simulink model "simulazione_006_s"  (R2016b)
settings: Solver=ode4  StartTime=0.0  StopTime=t_sim  FixedStep=step  RelTol=1e-3
values from neighbouring files (symbols this model uses):
  motion_time = 5    [simulazione_006_init.m]
  movement_lower_limit = -movement_upper_limit    [simulazione_006_init.m]
  movement_upper_limit = [2*pi; 2*pi; 2*pi; 2*pi; 2*pi; 2*pi]    [simulazione_006_init.m]
  p_init = direct_kinematic(q_init)    [simulazione_006_init.m]
  q_init = [pi/2; pi/3; -pi/9; pi/3; pi/5; pi/8]    [simulazione_006_init.m]
  radius = 0.1    [simulazione_006_init.m]
  ref_pulse = 2 * pi * frequency    (= 0.628318530718)    [simulazione_006_init.m]
  velocity_lower_limit = -velocity_upper_limit    [simulazione_006_init.m]
  velocity_upper_limit = [2*pi/3; 2*pi/3; pi; pi; pi; pi]    [simulazione_006_init.m]
settings Model: Creator=IBM  LastModifiedBy=IBM

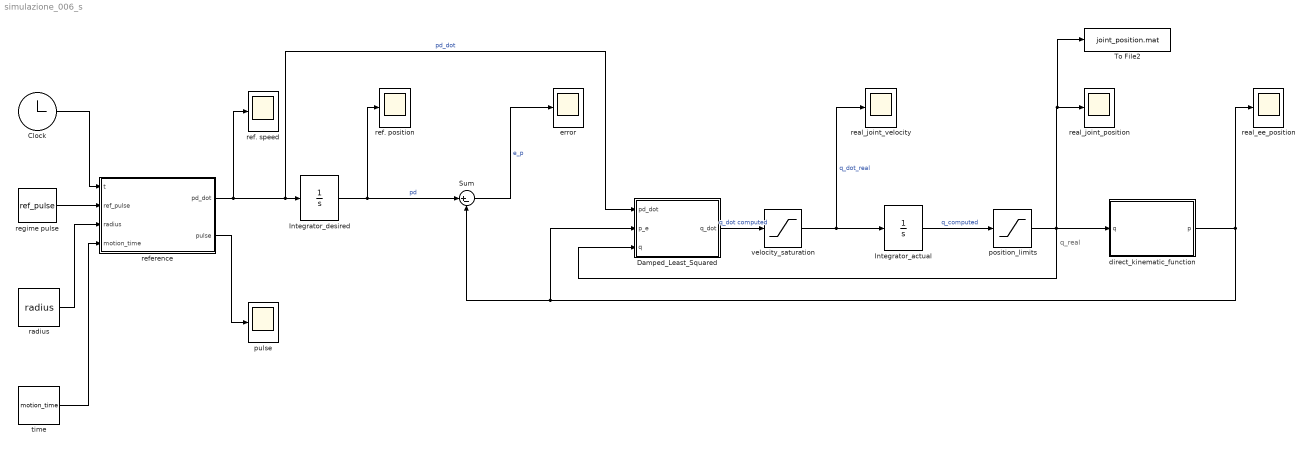
== system simulazione_006_s ==
  note: q_real
  Clock : Clock
  Damped_Least_Squared : MATLAB Function  TreatAsAtomicUnit=on
  Integrator_actual : Integrator  InitialCondition=q_init
  Integrator_desired : Integrator  InitialCondition=p_init
  Sum : Sum  Inputs=|+-
  To File2 : ToFile  Filename=joint_position.mat  MatrixName=q
  direct_kinematic_function : MATLAB Function  TreatAsAtomicUnit=on
  error : Scope
  position_limits : Saturate  UpperLimit=movement_upper_limit  LowerLimit=movement_lower_limit
  pulse : Scope
  radius : Constant  Value=radius
  real_ee_position : Scope
  real_joint_position : Scope
  real_joint_velocity : Scope
  ref. position : Scope
  ref. speed : Scope
  reference : MATLAB Function  TreatAsAtomicUnit=on
  regime pulse : Constant  Value=ref_pulse
  time : Constant  Value=motion_time
  velocity_saturation : Saturate  UpperLimit=velocity_upper_limit  LowerLimit=velocity_lower_limit
  wires:
  Clock/1 -> reference/1(t)
  Integrator_desired/1 -> ref. position/1, Sum/1  "pd"
  radius/1 -> reference/3(radius)
  Sum/1 -> error/1  "e_p"
  Integrator_actual/1 -> position_limits/1  "q_computed"
  direct_kinematic_function/1(p) -> real_ee_position/1, Damped_Least_Squared/2(p_e), Sum/2
  regime pulse/1 -> reference/2(ref_pulse)
  reference/1(pd_dot) -> ref. speed/1, Damped_Least_Squared/1(pd_dot), Integrator_desired/1  "pd_dot"
  time/1 -> reference/4(motion_time)
  reference/2(pulse) -> pulse/1
  Damped_Least_Squared/1(q_dot) -> velocity_saturation/1  "q_dot computed"
  velocity_saturation/1 -> real_joint_velocity/1, Integrator_actual/1  "q_dot_real"
  position_limits/1 -> Damped_Least_Squared/3(q), To File2/1, real_joint_position/1, direct_kinematic_function/1(q)

== matlab function simulazione_006_s/Damped_Least_Squared ==
  data: pd_dot input; p_e input; q_dot output; q input
function q_dot = dls(pd_dot, p_e, q)
    
    Jg = geometric_jacobian(q);
    Ja = analytic_jacobian(Jg, p_e);
    
    s = svd(Ja);
    sigma_th = 1/pi;
    sigma = s(6);
    lambda_max = 0.001;
    
    if sigma >= sigma_th 
        lambda = 0; 
    else
        lambda = lambda_max - lambda_max * sigma / sigma_th;
    end
    
    q_dot = transpose(Ja) * inv(Ja * transpose(Ja) + lambda * eye(6)) * pd_dot;
    
end

== matlab function simulazione_006_s/reference ==
  data: t input; ref_pulse input; pd_dot output; radius input; motion_time input; pulse output
function [pd_dot, pulse] = reference(t, ref_pulse, radius, motion_time)

    [pd_dot, pulse] = circular_reference(t, ref_pulse, radius, motion_time);
    
end

== matlab function simulazione_006_s/direct_kinematic_function ==
  data: q input; p output
function p = dkf(q)

    p = direct_kinematic(q);
